simulink model "dfig(1)"  (R2022b)
settings: Solver=VariableStepAuto  StartTime=0.0  StopTime=10.0  RelTol=1e-3
values from neighbouring files (symbols this model uses):
  Cbus = 80e-3    (= 0.08)    [dfigcode.m]
  D = 1e-3    (= 0.001)    [dfigcode.m]
  f = 50    [dfigcode.m]
  Fs = Vs*sqrt(2/3)/(2*pi*f)    [dfigcode.m]
  fsw = 4e3    (= 4000)    [dfigcode.m]
  J = 127/2    (= 63.5)    [dfigcode.m]
  ki_id = (wni^2)*Lr*sigma    (= 491.599501999)    [dfigcode.m]
  Ki_idg = (wnig^2)*Lg    (= 56.8489213503)    [dfigcode.m]
  ki_iq = ki_id    (= 491.599501999)    [dfigcode.m]
  Ki_iqg = Ki_idg    (= 56.8489213503)    [dfigcode.m]
  ki_n = ((wnn^2)*J)/p    (= 12700)    [dfigcode.m]
  Ki_v = -300000    [dfigcode.m]
  Kopt = ((0.5*ro*pi*(Radio^5)*Cp_max)/(lambda_opt^3))    (= 296454.198186)    [dfigcode.m]
  kp_id = (2*wni*sigma*Lr)-Rr    (= 0.5771)    [dfigcode.m]
  Kp_idg = (2*wnig*Lg)-Rg    (= 0.301572894745)    [dfigcode.m]
  kp_iq = kp_id    (= 0.5771)    [dfigcode.m]
  Kp_iqg = Kp_idg    (= 0.301572894745)    [dfigcode.m]
  kp_n = (2*wnn*J)/p    (= 1270)    [dfigcode.m]
  Kp_v = -1000    [dfigcode.m]
  Kpg = 1/(1.5*Vs*sqrt(2/3))    [dfigcode.m]
  Kqg = -Kpg    [dfigcode.m]
  Lg = 400e-6    (= 0.0004)    [dfigcode.m]
  Lm = 2.5e-3    (= 0.0025)    [dfigcode.m]
  Ls = Lm + Lsi    (= 0.002587)    [dfigcode.m]
  Lsi = 0.087e-3    (= 8.7e-05)    [dfigcode.m]
  N = 100    [dfigcode.m]
  n = 1500    [dfigcode.m]
  p = 2    [dfigcode.m]
  Ps = 2e6    (= 2000000)    [dfigcode.m]
  Rg = 20e-6    (= 2e-05)    [dfigcode.m]
  Rr = 2.9e-3    (= 0.0029)    [dfigcode.m]
  Rs = 2.6e-3    (= 0.0026)    [dfigcode.m]
  smax = 1/3    (= 0.333333333333)    [dfigcode.m]
  tab_lambda = (0.1:0.01:11.8)    [dfigcode.m]
  Tem = 12732    [dfigcode.m]
  Ts = 1/fsw/50    (= 5e-06)    [dfigcode.m]
  Vbus = 1150    [dfigcode.m]
  Vs = 690    [dfigcode.m]
undefined symbols (not defined in the file or in its folder): Ct, DiscIntNeverNeededParam
libraries: spsSeriesRLCBranchLib x4, spsThreePhaseVIMeasurementLib x3, spsPWMGenerator2LevelLib x2, spsUniversalBridgeLib x2, spsAsynchronousMachineSIUnitsLib x1, spsGroundLib x1, spsMultimeterLib x1, spsThreePhaseProgrammableVoltageSourceLib x1, spsThreePhaseTransformerTwoWindingsLib x1, sps_lib x1
settings Model: Creator=prithika  LastModifiedBy=prithika

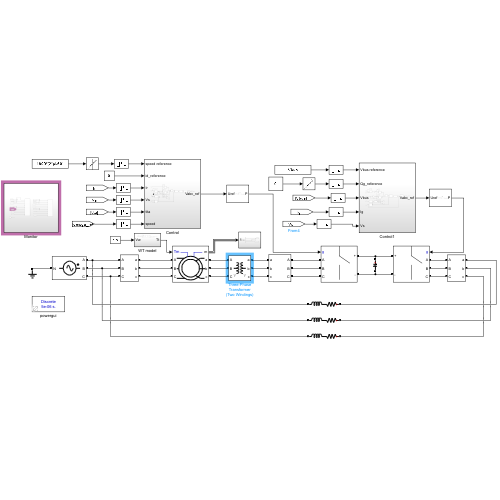
[thumbnail: Simulink's stored preview of the top-level diagram]
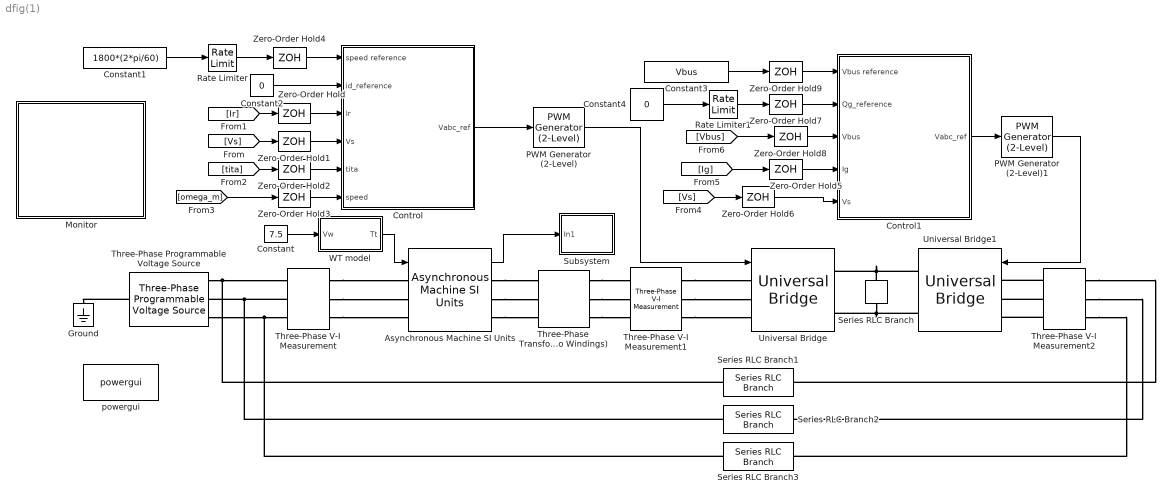
== system dfig(1) ==
  Asynchronous Machine SI Units : spsAsynchronousMachineSIUnitsLib/Asynchronous Machine SI Units  RotorType=Wound  PresetModel=No  MechanicalLoad=Torque Tm  ShowDetailedParameters=on  ReferenceFrame=Rotor  Units=SI  MeasurementBus=off  NominalParameters=[Ps Vs f]  VoltageRatio=1  Stator=[Rs , Lsi]  Rotor=[Rr , Lsi]  Cage1=[0.4155 0.002066]  Cage2=[0.4168 0.0003495]  Lm=Lm  Mechanical=[J D 2]  PolePairs=2  InitialConditions=[1 0 0 0 0 0 0 0]  SimulateSaturation=off  Saturation=[14.03593122, 27.81365428, 53.79336849, 72.68890987, 97.98006896, 148.6815601, 215.7428561, 302.9841135, 428.7778367 ; 230, 322, 414, 460, 506, 552, 598, 644, 690]  LoadFlowParameters=1492000  TsPowergui=0  TsBlock=-1  IterativeModel=Trapezoidal non iterative  IterativeDiscreteModel=Trapezoidal non iterative  Pmec=1.492e+006
  Constant : Constant  Value=7.5
  Constant1 : Constant  Value=1800*(2*pi/60)
  Constant2 : Constant  Value=0
  Constant3 : Constant  Value=Vbus
  Constant4 : Constant  Value=0
  Control : Subsystem
  Control1 : Subsystem
  Ground : spsGroundLib/Ground  LConnTagsString=a
  Monitor : Subsystem
  PWM Generator (2-Level) : spsPWMGenerator2LevelLib/PWM Generator (2-Level)  ModulatorType=Three-phase bridge (6 pulses)  ModulatorMode=Unsynchronized  Fc=fsw  Pc=0  nF=27  MinMax="[ -1  1 ]"  SamplingTechnique=Symmetrical regular (single edge)  ModulatingSignals=off  m=0.8  Freq=60  Phase=0  Ts=0  ShowCarrierOutport=off
  PWM Generator (2-Level)1 : spsPWMGenerator2LevelLib/PWM Generator (2-Level)  ModulatorType=Three-phase bridge (6 pulses)  ModulatorMode=Unsynchronized  Fc=fsw  Pc=0  nF=27  MinMax="[ -1  1 ]"  SamplingTechnique=Symmetrical regular (single edge)  ModulatingSignals=off  m=0.8  Freq=60  Phase=0  Ts=0  ShowCarrierOutport=off
  Rate Limiter : RateLimiter  RisingSlewLimit=100/1  FallingSlewLimit=-100/1  SampleTimeMode=inherited
  Rate Limiter1 : RateLimiter  RisingSlewLimit=1000e3/2  FallingSlewLimit=-1000e3/2  SampleTimeMode=inherited
  Series RLC Branch : spsSeriesRLCBranchLib/Series RLC Branch  LConnTagsString=__new0  RConnTagsString=__new0  BranchType=C  Resistance=1  Inductance=1e-3  SetiL0=off  InitialCurrent=0  Capacitance=Cbus  Setx0=on  InitialVoltage=0  Measurements=Branch voltage
  Series RLC Branch1 : spsSeriesRLCBranchLib/Series RLC Branch  LConnTagsString=__new0  RConnTagsString=__new0  BranchType=RL  Resistance=Rg  Inductance=Lg  SetiL0=off  InitialCurrent=0  Capacitance=Cbus  Setx0=on  InitialVoltage=0  Measurements=None
  Series RLC Branch2 : spsSeriesRLCBranchLib/Series RLC Branch  LConnTagsString=__new0  RConnTagsString=__new0  BranchType=RL  Resistance=Rg  Inductance=Lg  SetiL0=off  InitialCurrent=0  Capacitance=Cbus  Setx0=on  InitialVoltage=0  Measurements=None
  Series RLC Branch3 : spsSeriesRLCBranchLib/Series RLC Branch  LConnTagsString=__new0  RConnTagsString=__new0  BranchType=RL  Resistance=Rg  Inductance=Lg  SetiL0=off  InitialCurrent=0  Capacitance=Cbus  Setx0=on  InitialVoltage=0  Measurements=None
  Subsystem : Subsystem
  Three-Phase Programmable Voltage Source : spsThreePhaseProgrammableVoltageSourceLib/Three-Phase Programmable Voltage Source  PositiveSequence="[Vs  0 f]"  VariationEntity=None  VariationType=Table of time-amplitude pairs  VariationTypeAlt=Step  VariationStep=0.5  VariationRate=10  VariationMagnitude=0.3  VariationFrequency=2  VariationTiming=[1 2]  VariationPhaseA=off  Amplitudes=[1 0.8 1.2 1.0]  TimeValues=[0 0.1 0.15 0.2]  HarmonicGeneration=off  HarmonicA=[3 0.2 -25 0]  HarmonicB=[2 0.15 35 2]  Timing="[0.05  3]"  BusType=swing  Pref=0  Qref=0  Qmin=-inf  Qmax=inf
  Three-Phase Transformer (Two Windings) : spsThreePhaseTransformerTwoWindingsLib/Three-Phase Transformer (Two Windings)  Winding1Connection=Y  Winding2Connection=Y  CoreType=Three single-phase transformers  SetSaturation=off  Hysteresis=off  DataFile='hysteresis'  SetInitialFlux=off  Measurements=None  UNITS=SI  NominalPower=[ Ps , f ]  Winding1=[Vs 0 0]  Winding2=[Vs/u 0.0 0.0]  Rm=1.0804e+06  Lm=2866  L0=0.5  Saturation=[0 0;0.66653 1910.3;277.72 2419.7]  InitialFluxes=[ 0.8 , -0.8 , 0.7 ]  BreakLoop=off  DiscreteSolver=Trapezoidal iterative  DataType=on  TransfoNumber=1
  Three-Phase V-I Measurement : spsThreePhaseVIMeasurementLib/Three-Phase V-I Measurement  VoltageMeasurement=phase-to-ground  SetLabelV=on  LabelV=Vs  Vpu=off  VpuLL=off  CurrentMeasurement=yes  SetLabelI=on  LabelI=Is  Ipu=off  Pbase=100e6  Vbase=500e3  OutputType=Complex  PhasorSimulation=off  PSBequivalent=0
  Three-Phase V-I Measurement1 : spsThreePhaseVIMeasurementLib/Three-Phase V-I Measurement  VoltageMeasurement=no  SetLabelV=off  LabelV=Vs  Vpu=off  VpuLL=off  CurrentMeasurement=yes  SetLabelI=on  LabelI=Ir  Ipu=off  Pbase=100e6  Vbase=500e3  OutputType=Complex  PhasorSimulation=off  PSBequivalent=0
  Three-Phase V-I Measurement2 : spsThreePhaseVIMeasurementLib/Three-Phase V-I Measurement  VoltageMeasurement=no  SetLabelV=on  LabelV=Vs  Vpu=on  VpuLL=off  CurrentMeasurement=yes  SetLabelI=on  LabelI=Ig  Ipu=off  Pbase=100e6  Vbase=500e3  OutputType=Complex  PhasorSimulation=off  PSBequivalent=0
  Universal Bridge : spsUniversalBridgeLib/Universal Bridge  Arms=3  SnubberResistance=1e5  SnubberCapacitance=inf  Device=Ideal Switches  Ron=1e-3  Lon=0  ForwardVoltages="[  0  0  ]"  ForwardVoltage=0  GTOparameters=[ 10e-6 , 20e-6 ]  IGBTparameters=[ 1e-6 , 2e-6 ]  Measurements=None  Measurements_2=None  converterType=Rectifier
  Universal Bridge1 : spsUniversalBridgeLib/Universal Bridge  Arms=3  SnubberResistance=1e5  SnubberCapacitance=inf  Device=Ideal Switches  Ron=1e-3  Lon=0  ForwardVoltages="[  0  0  ]"  ForwardVoltage=0  GTOparameters=[ 10e-6 , 20e-6 ]  IGBTparameters=[ 1e-6 , 2e-6 ]  Measurements=None  Measurements_2=None  converterType=Rectifier
  WT model : Subsystem
  Zero-Order Hold{,1..9} (10 alike) : ZeroOrderHold  SampleTime=1/fsw
  powergui : sps_lib/powergui  Priority=1  SimulationMode=Discrete  SampleTime=Ts  frequency=60  Iterations=50  frequencyindice=50  Pbase=100e6  ErrMax=1e-4  UnitsV=kV  UnitsW=MW  buscounter=0  FunctionMessages=off  echomessages=off  EnableUseOfTLC=off  CurrentSourceSwitches=off  DisableSnubberDevices=off  DisableRonSwitches=off  DisableVfSwitches=off  DisplayEquations=off  AutomaticDiscreteSolvers=off  SolverType=Tustin/Backward Euler (TBE)  Interpol=off  ExternalGateDelay=off  methode=off  Ts=100  x0status=blocks  SPID=on  SwTol=0  HookPort=off  NonlinearTolerance=1e-4  nMaxIteration=100  ContinueOnMaxIteration=off  RestoreLinks=warning  ResistiveCurrentMeasurement=off  Frange=[0:2:500]  Ylog=off  Xlog=on  ShowGrid=off  save=off  variable=ZData  structure=0  ZoomFFT=off  StartTime=0.0  cycles=1  DisplayStyle=1  fundamental=60  FreqAxis=off  MaxFrequency=1000  frequencyindicesteady=1  RmsSteady=1  display=off
  wires:
  PWM Generator (2-Level)/1 -> Universal Bridge/1
  Control/1(Vabc_ref) -> PWM Generator (2-Level)/1
  Constant2/1 -> Control/2(id_reference)
  Constant1/1 -> Rate Limiter/1
  [Vs] -> Zero-Order Hold1/1
  [Ir] -> Zero-Order Hold/1
  Asynchronous Machine SI Units/1 -> Subsystem/1(In1)
  [tita] -> Zero-Order Hold2/1
  [omega_m] -> Zero-Order Hold3/1
  Zero-Order Hold/1 -> Control/3(Ir)
  Zero-Order Hold1/1 -> Control/4(Vs)
  Zero-Order Hold2/1 -> Control/5(tita)
  Zero-Order Hold3/1 -> Control/6(speed)
  Zero-Order Hold4/1 -> Control/1(speed reference)
  Rate Limiter/1 -> Zero-Order Hold4/1
  Constant/1 -> WT model/1(Vw)
  WT model/1(Tt) -> Asynchronous Machine SI Units/1
  PWM Generator (2-Level)1/1 -> Universal Bridge1/1
  Constant4/1 -> Rate Limiter1/1
  Zero-Order Hold9/1 -> Control1/1(Vbus reference)
  Constant3/1 -> Zero-Order Hold9/1
  [Vs] -> Zero-Order Hold6/1
  [Ig] -> Zero-Order Hold5/1
  Zero-Order Hold5/1 -> Control1/4(Ig)
  Zero-Order Hold6/1 -> Control1/5(Vs)
  Control1/1(Vabc_ref) -> PWM Generator (2-Level)1/1
  Zero-Order Hold7/1 -> Control1/2(Qg_reference)
  Rate Limiter1/1 -> Zero-Order Hold7/1
  [Vbus] -> Zero-Order Hold8/1
  Zero-Order Hold8/1 -> Control1/3(Vbus)
  connections:
  Three-Phase Programmable Voltage Source/LConn1 -- Ground/LConn1
  Three-Phase V-I Measurement1/LConn2 -- Universal Bridge/LConn2
  Three-Phase V-I Measurement1/LConn1 -- Universal Bridge/LConn1
  Three-Phase V-I Measurement1/LConn3 -- Universal Bridge/LConn3
  Three-Phase Programmable Voltage Source/RConn1 -- Series RLC Branch1/RConn1 -- Three-Phase V-I Measurement/LConn1
  Three-Phase V-I Measurement/LConn2 -- Series RLC Branch2/RConn1 -- Three-Phase Programmable Voltage Source/RConn2
  Three-Phase Programmable Voltage Source/RConn3 -- Series RLC Branch3/RConn1 -- Three-Phase V-I Measurement/LConn3
  Three-Phase V-I Measurement/RConn1 -- Asynchronous Machine SI Units/LConn1
  Three-Phase V-I Measurement/RConn2 -- Asynchronous Machine SI Units/LConn2
  Three-Phase V-I Measurement/RConn3 -- Asynchronous Machine SI Units/LConn3
  Universal Bridge1/RConn1 -- Series RLC Branch/LConn1 -- Universal Bridge/RConn1
  Universal Bridge1/RConn2 -- Series RLC Branch/RConn1 -- Universal Bridge/RConn2
  Three-Phase V-I Measurement2/LConn2 -- Universal Bridge1/LConn2
  Three-Phase V-I Measurement2/LConn1 -- Universal Bridge1/LConn1
  Three-Phase V-I Measurement2/LConn3 -- Universal Bridge1/LConn3
  Three-Phase V-I Measurement2/RConn1 -- Series RLC Branch1/LConn1
  Three-Phase V-I Measurement2/RConn2 -- Series RLC Branch2/LConn1
  Three-Phase V-I Measurement2/RConn3 -- Series RLC Branch3/LConn1
  Asynchronous Machine SI Units/RConn1 -- Three-Phase Transformer (Two Windings)/LConn1
  Three-Phase Transformer (Two Windings)/RConn1 -- Three-Phase V-I Measurement1/RConn1
  Asynchronous Machine SI Units/RConn2 -- Three-Phase Transformer (Two Windings)/LConn2
  Asynchronous Machine SI Units/RConn3 -- Three-Phase Transformer (Two Windings)/LConn3
  Three-Phase Transformer (Two Windings)/RConn2 -- Three-Phase V-I Measurement1/RConn2
  Three-Phase Transformer (Two Windings)/RConn3 -- Three-Phase V-I Measurement1/RConn3

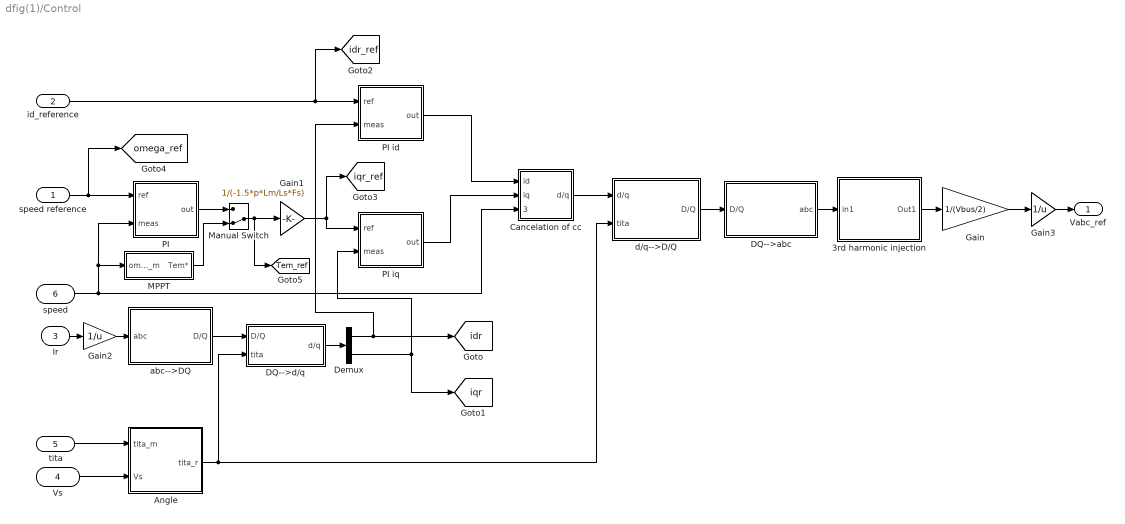
== system dfig(1)/Control ==
  speed reference : Inport
  id_reference : Inport  Port=2
  Ir : Inport  Port=3
  Vs : Inport  Port=4
  tita : Inport  Port=5
  speed : Inport  Port=6
  3rd harmonic injection : Subsystem
  Angle : Subsystem
  Cancelation of cc : Subsystem
  DQ-->abc : Subsystem
  DQ-->d/q : Subsystem
  Demux : Demux  Outputs=2
  Gain : Gain  Gain=1/(Vbus/2)
  Gain1 : Gain  Gain=1/(-1.5*p*Lm/Ls*Fs)
  Gain2 : Gain  Gain=1/u
  Gain3 : Gain  Gain=1/u
  MPPT : Subsystem
  Manual Switch : ManualSwitch  CurrentSetting=0
  "PI " : Subsystem
  PI id : Subsystem
  PI iq : Subsystem
  abc-->DQ : Subsystem
  d/q-->D/Q : Subsystem
  Vabc_ref : Outport
  tag scope: Tem_ref=global, idr=global, idr_ref=global, iqr=global, iqr_ref=global, omega_ref=global
  wires:
  DQ-->abc/1(abc) -> 3rd harmonic injection/1(in1)
  d/q-->D/Q/1(D/Q) -> DQ-->abc/1(D/Q)
  abc-->DQ/1(D/Q) -> DQ-->d/q/1(D/Q)
  3rd harmonic injection/1(Out1) -> Gain/1
  tita/1 -> Angle/1(tita_m)
  Vs/1 -> Angle/2(Vs)
  Angle/1(tita_r) -> d/q-->D/Q/2(tita), DQ-->d/q/2(tita)
  Cancelation of cc/1(d/q) -> d/q-->D/Q/1(d/q)
  PI id/1(out) -> Cancelation of cc/1(id)
  PI iq/1(out) -> Cancelation of cc/2(iq)
  speed/1 -> MPPT/1(omega_m), "PI "/2(meas), Cancelation of cc/3(omega)
  DQ-->d/q/1(d/q) -> Demux/1
  Demux/2 -> [iqr], PI iq/2(meas)
  Demux/1 -> [idr], PI id/2(meas)
  speed reference/1 -> [omega_ref], "PI "/1(ref)
  Gain1/1 -> [iqr_ref], PI iq/1(ref)
  id_reference/1 -> PI id/1(ref), [idr_ref]
  MPPT/1(Tem*) -> Manual Switch/2
  "PI "/1(out) -> Manual Switch/1
  Manual Switch/1 -> Gain1/1, [Tem_ref]
  Ir/1 -> Gain2/1
  Gain2/1 -> abc-->DQ/1(abc)
  Gain/1 -> Gain3/1
  Gain3/1 -> Vabc_ref/1

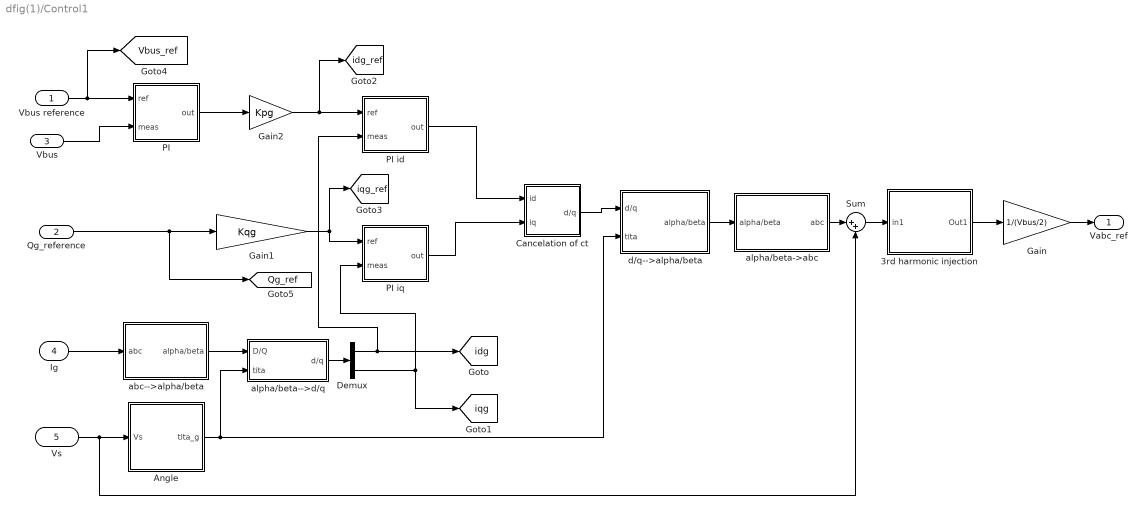
== system dfig(1)/Control1 ==
  Vbus reference : Inport
  Qg_reference : Inport  Port=2
  Vbus : Inport  Port=3
  Ig : Inport  Port=4
  Vs : Inport  Port=5
  3rd harmonic injection : Subsystem
  Angle : Subsystem
  Cancelation of ct : Subsystem
  Demux : Demux  Outputs=2
  Gain : Gain  Gain=1/(Vbus/2)
  Gain1 : Gain  Gain=Kqg
  Gain2 : Gain  Gain=Kpg
  "PI " : Subsystem
  PI id : Subsystem
  PI iq : Subsystem
  Sum : Sum  Inputs=|++
  abc-->alpha/beta : Subsystem
  alpha/beta-->d/q : Subsystem
  alpha/beta->abc : Subsystem
  d/q-->alpha/beta : Subsystem
  Vabc_ref : Outport
  tag scope: Qg_ref=global, Vbus_ref=global, idg=global, idg_ref=global, iqg=global, iqg_ref=global
  wires:
  Gain/1 -> Vabc_ref/1
  d/q-->alpha/beta/1(alpha/beta) -> alpha/beta->abc/1(alpha/beta)
  Ig/1 -> abc-->alpha/beta/1(abc)
  abc-->alpha/beta/1(alpha/beta) -> alpha/beta-->d/q/1(D/Q)
  3rd harmonic injection/1(Out1) -> Gain/1
  Vs/1 -> Sum/2, Angle/1(Vs)
  Angle/1(tita_g) -> d/q-->alpha/beta/2(tita), alpha/beta-->d/q/2(tita)
  Cancelation of ct/1(d/q) -> d/q-->alpha/beta/1(d/q)
  PI id/1(out) -> Cancelation of ct/1(id)
  PI iq/1(out) -> Cancelation of ct/2(iq)
  alpha/beta-->d/q/1(d/q) -> Demux/1
  Demux/2 -> [iqg], PI iq/2(meas)
  Demux/1 -> [idg], PI id/2(meas)
  Vbus reference/1 -> "PI "/1(ref), [Vbus_ref]
  Gain1/1 -> [iqg_ref], PI iq/1(ref)
  Qg_reference/1 -> Gain1/1, [Qg_ref]
  "PI "/1(out) -> Gain2/1
  Gain2/1 -> [idg_ref], PI id/1(ref)
  Vbus/1 -> "PI "/2(meas)
  alpha/beta->abc/1(abc) -> Sum/1
  Sum/1 -> 3rd harmonic injection/1(in1)

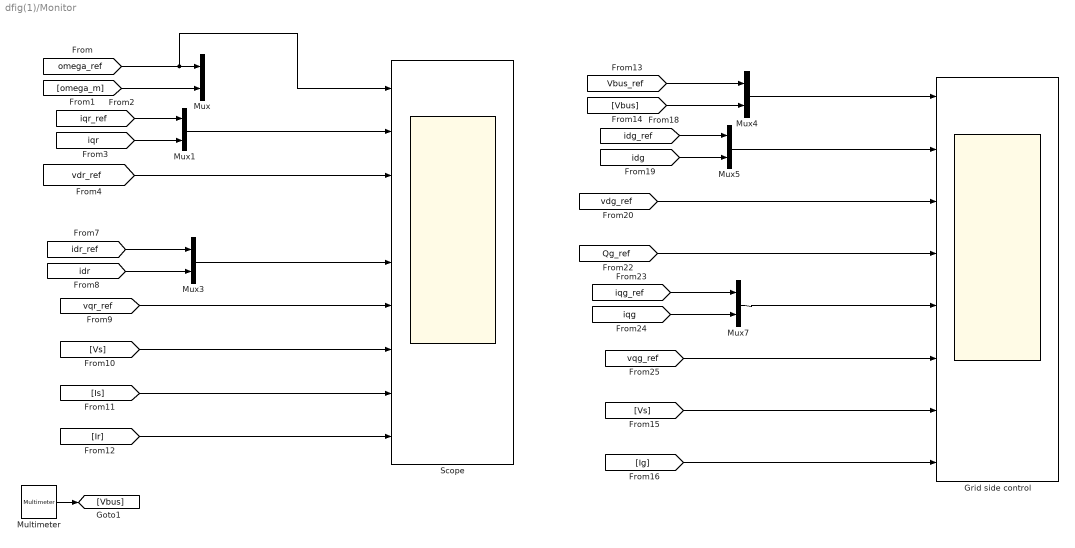
== system dfig(1)/Monitor ==
  Grid side control : Scope  NumInputPorts=8
  Multimeter : spsMultimeterLib/Multimeter  L=1  sel=1  yselected={}  Gain=0  OutputType=Complex  PlotAtSimulationStop=off  PhasorSimulation=off
  Mux{,1,3..5,7} (6 alike) : Mux  Inputs=2
  Scope : Scope  NumInputPorts=9
  wires:
  [omega_ref] -> Scope/1, Mux/1
  [omega_m] -> Mux/2
  [iqr_ref] -> Mux1/1
  [iqr] -> Mux1/2
  Mux1/1 -> Scope/2
  [vdr_ref] -> Scope/3
  [idr_ref] -> Mux3/1
  [idr] -> Mux3/2
  Mux3/1 -> Scope/5
  [Vs] -> Scope/7
  [Is] -> Scope/8
  [Ir] -> Scope/9
  [vqr_ref] -> Scope/6
  Multimeter/1 -> [Vbus]
  [Qg_ref] -> Grid side control/4
  [vqg_ref] -> Grid side control/6
  [vdg_ref] -> Grid side control/3
  [iqg] -> Mux7/2
  [iqg_ref] -> Mux7/1
  [Vbus_ref] -> Mux4/1
  [Vbus] -> Mux4/2
  [Ig] -> Grid side control/8
  [Vs] -> Grid side control/7
  Mux5/1 -> Grid side control/2
  [idg_ref] -> Mux5/1
  [idg] -> Mux5/2
  Mux7/1 -> Grid side control/5
  Mux4/1 -> Grid side control/1

== system dfig(1)/Subsystem ==
  In1 : Inport
  Bus Selector : BusSelector  OutputSignals=Mechanical.Rotor angle thetam (rad),Mechanical.Rotor speed (wm),Mechanical.Electromagnetic torque Te (N*m)
  wires:
  In1/1 -> Bus Selector/1
  Bus Selector/2 -> [omega_m]  "<Rotor speed (wm)>"
  Bus Selector/1 -> [tita]  "<Rotor angle thetam (rad)>"
  Bus Selector/3 -> [Tem]  "<Electromagnetic torque Te (N*m)>"

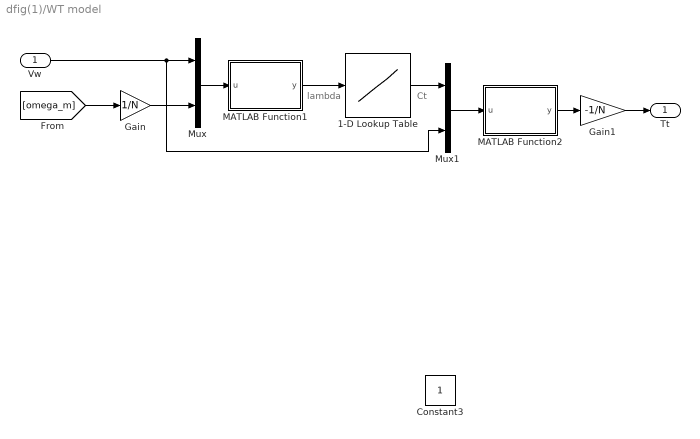
== system dfig(1)/WT model ==
  note: Ct
  note: lambda
  Vw : Inport
  1-D Lookup Table : Lookup_n-D  NumberOfTableDimensions=1  BreakpointsForDimension1=tab_lambda  BreakpointsForDimension1DataTypeStr=Inherit: Inherit from 'Breakpoint data'  Table=Ct  TableDataTypeStr=Inherit: Inherit from 'Table data'  InternalRulePriority=Speed  RndMeth=Simplest
  Constant3 : Constant
  Gain : Gain  Gain=1/N
  Gain1 : Gain  Gain=-1/N
  MATLAB Function1 : MATLAB Function  TreatAsAtomicUnit=on
  MATLAB Function2 : MATLAB Function  TreatAsAtomicUnit=on
  Mux : Mux  Inputs=2
  Mux1 : Mux  Inputs=2
  Tt : Outport
  wires:
  Vw/1 -> Mux1/2, Mux/1
  [omega_m] -> Gain/1
  Gain/1 -> Mux/2
  Mux/1 -> MATLAB Function1/1(u)
  MATLAB Function1/1(y) -> 1-D Lookup Table/1
  MATLAB Function2/1(y) -> Gain1/1
  Gain1/1 -> Tt/1
  1-D Lookup Table/1 -> Mux1/1
  Mux1/1 -> MATLAB Function2/1(u)

== system dfig(1)/Control/3rd harmonic injection ==
  in1 : Inport
  Gain : Gain  Gain=-0.5
  Max1 : MinMax  Function=max
  Min1 : MinMax
  Sum : Sum  Inputs=|++
  Sum1 : Sum  Inputs=|++
  Out1 : Outport
  wires:
  in1/1 -> Max1/1, Min1/1, Sum/1
  Sum/1 -> Out1/1
  Min1/1 -> Sum1/1
  Sum1/1 -> Gain/1
  Gain/1 -> Sum/2
  Max1/1 -> Sum1/2

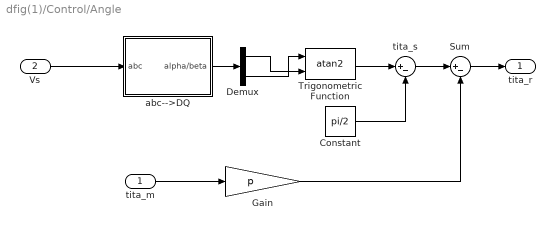
== system dfig(1)/Control/Angle ==
  tita_m : Inport
  Vs : Inport  Port=2
  Constant : Constant  Value=pi/2
  Demux : Demux  Outputs=2
  Gain : Gain  Gain=p
  Sum : Sum  Inputs=|+-
  Trigonometric Function : Trigonometry  Operator=atan2
  abc-->DQ : Subsystem
  tita_s : Sum  Inputs=|+-
  tita_r : Outport
  wires:
  Vs/1 -> abc-->DQ/1(abc)
  abc-->DQ/1(alpha/beta) -> Demux/1
  Demux/1 -> Trigonometric Function/2
  Demux/2 -> Trigonometric Function/1
  Trigonometric Function/1 -> tita_s/1
  Constant/1 -> tita_s/2
  tita_m/1 -> Gain/1
  tita_s/1 -> Sum/1
  Sum/1 -> tita_r/1
  Gain/1 -> Sum/2

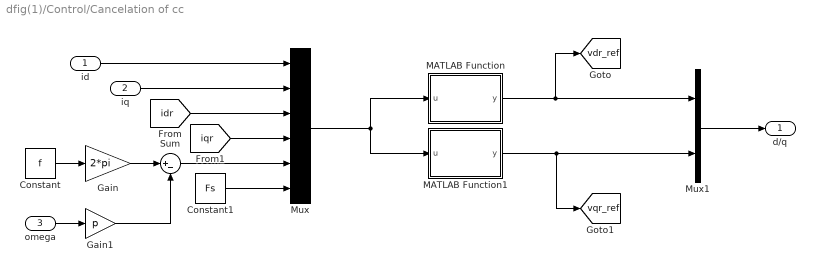
== system dfig(1)/Control/Cancelation of cc ==
  id : Inport
  iq : Inport  Port=2
  omega : Inport  Port=3
  Constant : Constant  Value=f
  Constant1 : Constant  Value=Fs
  Gain : Gain  Gain=2*pi
  Gain1 : Gain  Gain=p
  MATLAB Function : MATLAB Function  TreatAsAtomicUnit=on
  MATLAB Function1 : MATLAB Function  TreatAsAtomicUnit=on
  Mux : Mux  Inputs=6
  Mux1 : Mux  Inputs=2
  Sum : Sum  Inputs=|+-
  d/q : Outport
  tag scope: vdr_ref=global, vqr_ref=global
  wires:
  id/1 -> Mux/1
  iq/1 -> Mux/2
  [idr] -> Mux/3
  [iqr] -> Mux/4
  Constant/1 -> Gain/1
  Gain/1 -> Sum/1
  Sum/1 -> Mux/5
  Constant1/1 -> Mux/6
  omega/1 -> Gain1/1
  Gain1/1 -> Sum/2
  Mux/1 -> MATLAB Function/1(u), MATLAB Function1/1(u)
  MATLAB Function/1(y) -> [vdr_ref], Mux1/1
  MATLAB Function1/1(y) -> [vqr_ref], Mux1/2
  Mux1/1 -> d/q/1

== system dfig(1)/Control/DQ-->abc ==
  D/Q : Inport
  MATLAB Function : MATLAB Function  TreatAsAtomicUnit=on
  MATLAB Function1 : MATLAB Function  TreatAsAtomicUnit=on
  MATLAB Function2 : MATLAB Function  TreatAsAtomicUnit=on
  Mux : Mux  Inputs=3
  abc : Outport
  wires:
  MATLAB Function/1(y) -> Mux/1
  MATLAB Function1/1(y) -> Mux/2
  MATLAB Function2/1(y) -> Mux/3
  D/Q/1 -> MATLAB Function2/1(u), MATLAB Function1/1(u), MATLAB Function/1(u)
  Mux/1 -> abc/1

== system dfig(1)/Control/DQ-->d//q ==
  D/Q : Inport
  tita : Inport  Port=2
  MATLAB Function : MATLAB Function  TreatAsAtomicUnit=on
  MATLAB Function1 : MATLAB Function  TreatAsAtomicUnit=on
  Mux : Mux  Inputs=2
  Mux1 : Mux  Inputs=2
  d/q : Outport
  wires:
  D/Q/1 -> Mux/1
  tita/1 -> Mux/2
  Mux/1 -> MATLAB Function1/1(u), MATLAB Function/1(u)
  MATLAB Function/1(y) -> Mux1/1
  MATLAB Function1/1(y) -> Mux1/2
  Mux1/1 -> d/q/1

== system dfig(1)/Control/MPPT ==
  omega_m : Inport
  Gain : Gain  Gain=1/N
  Gain1 : Gain  Gain=-Kopt
  Gain2 : Gain  Gain=1/n
  MATLAB Function : MATLAB Function  TreatAsAtomicUnit=on
  Tem* : Outport
  wires:
  MATLAB Function/1(y) -> Gain1/1
  omega_m/1 -> Gain/1
  Gain/1 -> MATLAB Function/1(u)
  Gain1/1 -> Gain2/1
  Gain2/1 -> Tem*/1

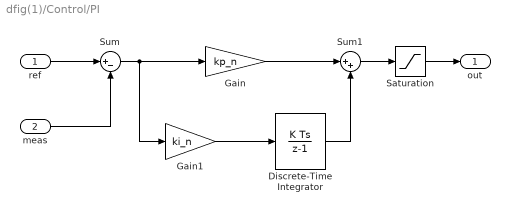
== system dfig(1)/Control/PI  ==
  ref : Inport
  meas : Inport  Port=2
  Discrete-Time Integrator : DiscreteIntegrator  SampleTime=1/fsw  LimitOutput=on  UpperSaturationLimit=Tem  LowerSaturationLimit=-Tem  ICPrevOutput=DiscIntNeverNeededParam  ICPrevScaledInput=DiscIntNeverNeededParam
  Gain : Gain  Gain=kp_n
  Gain1 : Gain  Gain=ki_n
  Saturation : Saturate  UpperLimit=Tem  LowerLimit=-Tem
  Sum : Sum  Inputs=|+-
  Sum1 : Sum  Inputs=|++
  out : Outport
  wires:
  Gain1/1 -> Discrete-Time Integrator/1
  Sum1/1 -> Saturation/1
  ref/1 -> Sum/1
  meas/1 -> Sum/2
  Sum/1 -> Gain1/1, Gain/1
  Gain/1 -> Sum1/1
  Discrete-Time Integrator/1 -> Sum1/2
  Saturation/1 -> out/1

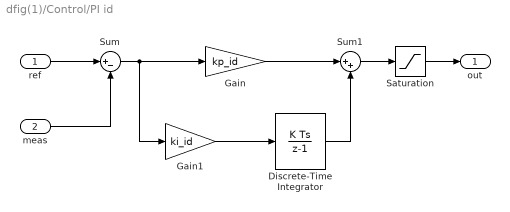
== system dfig(1)/Control/PI id ==
  ref : Inport
  meas : Inport  Port=2
  Discrete-Time Integrator : DiscreteIntegrator  SampleTime=1/fsw  LimitOutput=on  UpperSaturationLimit=Vbus/sqrt(3)  LowerSaturationLimit=-Vbus/sqrt(3)  ICPrevOutput=DiscIntNeverNeededParam  ICPrevScaledInput=DiscIntNeverNeededParam
  Gain : Gain  Gain=kp_id
  Gain1 : Gain  Gain=ki_id
  Saturation : Saturate  UpperLimit=Vbus/sqrt(3)  LowerLimit=-Vbus/sqrt(3)
  Sum : Sum  Inputs=|+-
  Sum1 : Sum  Inputs=|++
  out : Outport
  wires:
  Gain1/1 -> Discrete-Time Integrator/1
  Sum1/1 -> Saturation/1
  ref/1 -> Sum/1
  meas/1 -> Sum/2
  Sum/1 -> Gain1/1, Gain/1
  Gain/1 -> Sum1/1
  Discrete-Time Integrator/1 -> Sum1/2
  Saturation/1 -> out/1

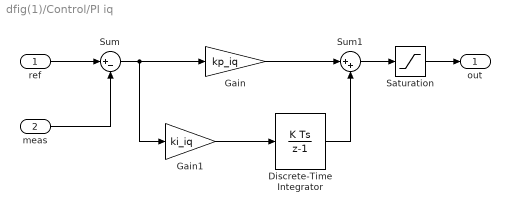
== system dfig(1)/Control/PI iq ==
  ref : Inport
  meas : Inport  Port=2
  Discrete-Time Integrator : DiscreteIntegrator  SampleTime=1/fsw  LimitOutput=on  UpperSaturationLimit=Vbus/sqrt(3)  LowerSaturationLimit=-Vbus/sqrt(3)  ICPrevOutput=DiscIntNeverNeededParam  ICPrevScaledInput=DiscIntNeverNeededParam
  Gain : Gain  Gain=kp_iq
  Gain1 : Gain  Gain=ki_iq
  Saturation : Saturate  UpperLimit=Vbus/sqrt(3)  LowerLimit=-Vbus/sqrt(3)
  Sum : Sum  Inputs=|+-
  Sum1 : Sum  Inputs=|++
  out : Outport
  wires:
  Gain1/1 -> Discrete-Time Integrator/1
  Sum1/1 -> Saturation/1
  ref/1 -> Sum/1
  meas/1 -> Sum/2
  Sum/1 -> Gain1/1, Gain/1
  Gain/1 -> Sum1/1
  Discrete-Time Integrator/1 -> Sum1/2
  Saturation/1 -> out/1

== system dfig(1)/Control/abc-->DQ ==
  abc : Inport
  MATLAB Function : MATLAB Function  TreatAsAtomicUnit=on
  MATLAB Function1 : MATLAB Function  TreatAsAtomicUnit=on
  Mux : Mux  Inputs=2
  D/Q : Outport
  wires:
  abc/1 -> MATLAB Function1/1(u), MATLAB Function/1(u)
  MATLAB Function/1(y) -> Mux/1
  MATLAB Function1/1(y) -> Mux/2
  Mux/1 -> D/Q/1

== system dfig(1)/Control/d//q-->D//Q ==
  d/q : Inport
  tita : Inport  Port=2
  MATLAB Function : MATLAB Function  TreatAsAtomicUnit=on
  MATLAB Function1 : MATLAB Function  TreatAsAtomicUnit=on
  Mux : Mux  Inputs=2
  Mux1 : Mux  Inputs=2
  D/Q : Outport
  wires:
  d/q/1 -> Mux/1
  tita/1 -> Mux/2
  Mux/1 -> MATLAB Function1/1(u), MATLAB Function/1(u)
  MATLAB Function/1(y) -> Mux1/1
  MATLAB Function1/1(y) -> Mux1/2
  Mux1/1 -> D/Q/1

== system dfig(1)/Control1/3rd harmonic injection ==
  in1 : Inport
  Gain : Gain  Gain=-0.5
  Max1 : MinMax  Function=max
  Min1 : MinMax
  Sum : Sum  Inputs=|++
  Sum1 : Sum  Inputs=|++
  Out1 : Outport
  wires:
  in1/1 -> Max1/1, Min1/1, Sum/1
  Sum/1 -> Out1/1
  Min1/1 -> Sum1/1
  Sum1/1 -> Gain/1
  Gain/1 -> Sum/2
  Max1/1 -> Sum1/2

== system dfig(1)/Control1/Angle ==
  note: tita_g
  Vs : Inport
  Demux : Demux  Outputs=2
  Trigonometric Function : Trigonometry  Operator=atan2
  abc-->alpha/beta : Subsystem
  tita_g : Outport
  wires:
  Vs/1 -> abc-->alpha/beta/1(abc)
  abc-->alpha/beta/1(alpha/beta) -> Demux/1
  Demux/1 -> Trigonometric Function/2
  Demux/2 -> Trigonometric Function/1
  Trigonometric Function/1 -> tita_g/1

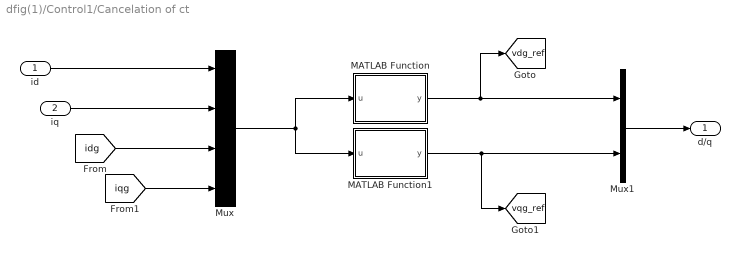
== system dfig(1)/Control1/Cancelation of ct ==
  id : Inport
  iq : Inport  Port=2
  MATLAB Function : MATLAB Function  TreatAsAtomicUnit=on
  MATLAB Function1 : MATLAB Function  TreatAsAtomicUnit=on
  Mux : Mux
  Mux1 : Mux  Inputs=2
  d/q : Outport
  tag scope: vdg_ref=global, vqg_ref=global
  wires:
  id/1 -> Mux/1
  iq/1 -> Mux/2
  [idg] -> Mux/3
  [iqg] -> Mux/4
  Mux/1 -> MATLAB Function/1(u), MATLAB Function1/1(u)
  MATLAB Function/1(y) -> [vdg_ref], Mux1/1
  MATLAB Function1/1(y) -> [vqg_ref], Mux1/2
  Mux1/1 -> d/q/1

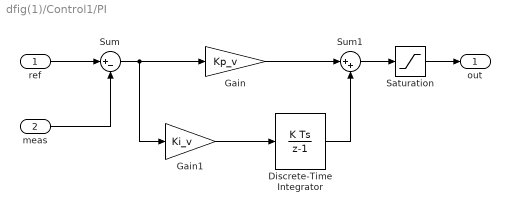
== system dfig(1)/Control1/PI  ==
  ref : Inport
  meas : Inport  Port=2
  Discrete-Time Integrator : DiscreteIntegrator  SampleTime=1/fsw  LimitOutput=on  UpperSaturationLimit=Ps*smax  LowerSaturationLimit=-Ps*smax  ICPrevOutput=DiscIntNeverNeededParam  ICPrevScaledInput=DiscIntNeverNeededParam
  Gain : Gain  Gain=Kp_v
  Gain1 : Gain  Gain=Ki_v
  Saturation : Saturate  UpperLimit=Ps*smax  LowerLimit=-Ps*smax
  Sum : Sum  Inputs=|+-
  Sum1 : Sum  Inputs=|++
  out : Outport
  wires:
  Gain1/1 -> Discrete-Time Integrator/1
  Sum1/1 -> Saturation/1
  ref/1 -> Sum/1
  meas/1 -> Sum/2
  Sum/1 -> Gain1/1, Gain/1
  Gain/1 -> Sum1/1
  Discrete-Time Integrator/1 -> Sum1/2
  Saturation/1 -> out/1

== system dfig(1)/Control1/PI id ==
  ref : Inport
  meas : Inport  Port=2
  Discrete-Time Integrator : DiscreteIntegrator  SampleTime=1/fsw  LimitOutput=on  UpperSaturationLimit=Vbus/sqrt(3)  LowerSaturationLimit=-Vbus/sqrt(3)  ICPrevOutput=DiscIntNeverNeededParam  ICPrevScaledInput=DiscIntNeverNeededParam
  Gain : Gain  Gain=Kp_idg
  Gain1 : Gain  Gain=Ki_idg
  Saturation : Saturate  UpperLimit=Vbus/sqrt(3)  LowerLimit=-Vbus/sqrt(3)
  Sum : Sum  Inputs=|+-
  Sum1 : Sum  Inputs=|++
  out : Outport
  wires:
  Gain1/1 -> Discrete-Time Integrator/1
  Sum1/1 -> Saturation/1
  ref/1 -> Sum/1
  meas/1 -> Sum/2
  Sum/1 -> Gain1/1, Gain/1
  Gain/1 -> Sum1/1
  Discrete-Time Integrator/1 -> Sum1/2
  Saturation/1 -> out/1

== system dfig(1)/Control1/PI iq ==
  ref : Inport
  meas : Inport  Port=2
  Discrete-Time Integrator : DiscreteIntegrator  SampleTime=1/fsw  LimitOutput=on  UpperSaturationLimit=Vbus/sqrt(3)  LowerSaturationLimit=-Vbus/sqrt(3)  ICPrevOutput=DiscIntNeverNeededParam  ICPrevScaledInput=DiscIntNeverNeededParam
  Gain : Gain  Gain=Kp_iqg
  Gain1 : Gain  Gain=Ki_iqg
  Saturation : Saturate  UpperLimit=Vbus/sqrt(3)  LowerLimit=-Vbus/sqrt(3)
  Sum : Sum  Inputs=|+-
  Sum1 : Sum  Inputs=|++
  out : Outport
  wires:
  Gain1/1 -> Discrete-Time Integrator/1
  Sum1/1 -> Saturation/1
  ref/1 -> Sum/1
  meas/1 -> Sum/2
  Sum/1 -> Gain1/1, Gain/1
  Gain/1 -> Sum1/1
  Discrete-Time Integrator/1 -> Sum1/2
  Saturation/1 -> out/1

== system dfig(1)/Control1/abc-->alpha//beta ==
  abc : Inport
  MATLAB Function : MATLAB Function  TreatAsAtomicUnit=on
  MATLAB Function1 : MATLAB Function  TreatAsAtomicUnit=on
  Mux : Mux  Inputs=2
  alpha/beta : Outport
  wires:
  abc/1 -> MATLAB Function1/1(u), MATLAB Function/1(u)
  MATLAB Function/1(y) -> Mux/1
  MATLAB Function1/1(y) -> Mux/2
  Mux/1 -> alpha/beta/1

== system dfig(1)/Control1/alpha//beta-->d//q ==
  D/Q : Inport
  tita : Inport  Port=2
  MATLAB Function : MATLAB Function  TreatAsAtomicUnit=on
  MATLAB Function1 : MATLAB Function  TreatAsAtomicUnit=on
  Mux : Mux  Inputs=2
  Mux1 : Mux  Inputs=2
  d/q : Outport
  wires:
  D/Q/1 -> Mux/1
  tita/1 -> Mux/2
  Mux/1 -> MATLAB Function1/1(u), MATLAB Function/1(u)
  MATLAB Function/1(y) -> Mux1/1
  MATLAB Function1/1(y) -> Mux1/2
  Mux1/1 -> d/q/1

== system dfig(1)/Control1/alpha//beta->abc ==
  alpha/beta : Inport
  MATLAB Function : MATLAB Function  TreatAsAtomicUnit=on
  MATLAB Function1 : MATLAB Function  TreatAsAtomicUnit=on
  MATLAB Function2 : MATLAB Function  TreatAsAtomicUnit=on
  Mux : Mux  Inputs=3
  abc : Outport
  wires:
  MATLAB Function/1(y) -> Mux/1
  MATLAB Function1/1(y) -> Mux/2
  MATLAB Function2/1(y) -> Mux/3
  alpha/beta/1 -> MATLAB Function2/1(u), MATLAB Function1/1(u), MATLAB Function/1(u)
  Mux/1 -> abc/1

== system dfig(1)/Control1/d//q-->alpha//beta ==
  d/q : Inport
  tita : Inport  Port=2
  MATLAB Function : MATLAB Function  TreatAsAtomicUnit=on
  MATLAB Function1 : MATLAB Function  TreatAsAtomicUnit=on
  Mux : Mux  Inputs=2
  Mux1 : Mux  Inputs=2
  alpha/beta : Outport
  wires:
  d/q/1 -> Mux/1
  tita/1 -> Mux/2
  Mux/1 -> MATLAB Function1/1(u), MATLAB Function/1(u)
  MATLAB Function/1(y) -> Mux1/1
  MATLAB Function1/1(y) -> Mux1/2
  Mux1/1 -> alpha/beta/1

== system dfig(1)/Control/Angle/abc-->DQ ==
  abc : Inport
  MATLAB Function : MATLAB Function  TreatAsAtomicUnit=on
  MATLAB Function1 : MATLAB Function  TreatAsAtomicUnit=on
  Mux : Mux  Inputs=2
  alpha/beta : Outport
  wires:
  abc/1 -> MATLAB Function1/1(u), MATLAB Function/1(u)
  MATLAB Function/1(y) -> Mux/1
  MATLAB Function1/1(y) -> Mux/2
  Mux/1 -> alpha/beta/1

== system dfig(1)/Control1/Angle/abc-->alpha//beta ==
  abc : Inport
  MATLAB Function : MATLAB Function  TreatAsAtomicUnit=on
  MATLAB Function1 : MATLAB Function  TreatAsAtomicUnit=on
  Mux : Mux  Inputs=2
  alpha/beta : Outport
  wires:
  abc/1 -> MATLAB Function1/1(u), MATLAB Function/1(u)
  MATLAB Function/1(y) -> Mux/1
  MATLAB Function1/1(y) -> Mux/2
  Mux/1 -> alpha/beta/1

== matlab function dfig(1)/WT model/MATLAB Function1 ==
  data: u input; y output
function y = fcn(u)
Radio = 42;
y = Radio * (u(2)/u(1))

== matlab function dfig(1)/Control1/Angle/abc-->alpha//beta/MATLAB Function ==
  data: u input; y output
function y = fcn(u)
y=(2/3) * (u(1) - u(2)/2 - u(3)/2);

== matlab function dfig(1)/Control/MPPT/MATLAB Function ==
  data: u input; y output
function y = fcn(u)

y = u(1)*u(1);

== matlab function dfig(1)/Control1/Angle/abc-->alpha//beta/MATLAB Function1 ==
  data: u input; y output
function y = fcn(u)

y=(2/3) * (u(2) * (sqrt(3)/2) - u(3) * (sqrt(3)/2));

== matlab function dfig(1)/Control1/Cancelation of ct/MATLAB Function ==
  data: u input; y output
function y = fcn(u)
Lg = 4.0000e-04;
f = 50;
y = u(1)-u(4)*Lg*(2*pi*f);

== matlab function dfig(1)/Control/DQ-->abc/MATLAB Function ==
  data: u input; y output
function y = fcn(u)
y=u(1);

== matlab function dfig(1)/Control1/Cancelation of ct/MATLAB Function1 ==
  data: u input; y output
function y = fcn(u)
Lg = 40000e-04;
f = 50;
y = u(2)+u(3)*Lg*(2*pi*f);

== matlab function dfig(1)/Control1/alpha//beta->abc/MATLAB Function ==
  data: u input; y output
function y = fcn(u)
y=u(1);

== matlab function dfig(1)/Control1/alpha//beta->abc/MATLAB Function1 ==
  data: u input; y output
function y = fcn(u)
y=-(u(1)/2)+u(2)*(sqrt(3)/2);

== matlab function dfig(1)/Control1/alpha//beta->abc/MATLAB Function2 ==
  data: u input; y output
function y = fcn(u)
y=-(u(1)/2)-u(2)*(sqrt(3)/2);

== matlab function dfig(1)/Control1/abc-->alpha//beta/MATLAB Function ==
  data: u input; y output
function y = fcn(u)

y = (2/3) * (u(1)-u(2)/2-u(3)/2);

== matlab function dfig(1)/Control1/abc-->alpha//beta/MATLAB Function1 ==
  data: u input; y output
function y = fcn(u)

y = (2/3) * (u(2)*(sqrt(3)/2)-u(3)*(sqrt(3)/2));

== matlab function dfig(1)/Control1/d//q-->alpha//beta/MATLAB Function ==
  data: u input; y output
function y = fcn(u)
y=u(1)*cos(u(3))-u(2)*sin(u(3));

== matlab function dfig(1)/Control1/d//q-->alpha//beta/MATLAB Function1 ==
  data: u input; y output
function y = fcn(u)
y=u(1)*sin(u(3))+u(2)*cos(u(3));

== matlab function dfig(1)/Control1/alpha//beta-->d//q/MATLAB Function ==
  data: u input; y output
function y = fcn(u)

y = u(1)*cos(u(3))+u(2)*sin(u(3));

== matlab function dfig(1)/Control1/alpha//beta-->d//q/MATLAB Function1 ==
  data: u input; y output
function y = fcn(u)

y = -u(1)*sin(u(3))+u(2)*cos(u(3));

== matlab function dfig(1)/Control/DQ-->abc/MATLAB Function2 ==
  data: u input; y output
function y = fcn(u)
y=-(u(1)/2)-u(2)*(sqrt(3)/2);

== matlab function dfig(1)/Control/d//q-->D//Q/MATLAB Function ==
  data: u input; y output
function y = fcn(u)
y=u(1)*cos(u(3))-u(2)*sin(u(3));

== matlab function dfig(1)/Control/d//q-->D//Q/MATLAB Function1 ==
  data: u input; y output
function y = fcn(u)
y=u(1)*sin(u(3))+u(2)*cos(u(3));

== matlab function dfig(1)/Control/DQ-->d//q/MATLAB Function ==
  data: u input; y output
function y = fcn(u)

y = u(1)*cos(u(3))+u(2)*sin(u(3));

== matlab function dfig(1)/Control/DQ-->d//q/MATLAB Function1 ==
  data: u input; y output
function y = fcn(u)

y = -u(1)*sin(u(3))+u(2)*cos(u(3));

== matlab function dfig(1)/Control/abc-->DQ/MATLAB Function ==
  data: u input; y output
function y = fcn(u)

y = (2/3) * (u(1)-u(2)/2-u(3)/2);

== matlab function dfig(1)/Control/abc-->DQ/MATLAB Function1 ==
  data: u input; y output
function y = fcn(u)

y = (2/3) * (u(2)*(sqrt(3)/2)-u(3)*(sqrt(3)/2));

== matlab function dfig(1)/Control/DQ-->abc/MATLAB Function1 ==
  data: u input; y output
function y = fcn(u)
y=-(u(1)/2)+u(2)*(sqrt(3)/2);

== matlab function dfig(1)/Control/Angle/abc-->DQ/MATLAB Function ==
  data: u input; y output
function y = fcn(u)
y=(2/3) * (u(1) - u(2)/2 - u(3)/2);

== matlab function dfig(1)/Control/Angle/abc-->DQ/MATLAB Function1 ==
  data: u input; y output
function y = fcn(u)

y=(2/3) * (u(2) * (sqrt(3)/2) - u(3) * (sqrt(3)/2));

== matlab function dfig(1)/Control/Cancelation of cc/MATLAB Function ==
  data: u input; y output
function y = fcn(u)
Lsi = 0.087e-3;
Lm = 2.5e-3;
Ls = Lm + Lsi;
Lr = Lm + Lsi;
sigma = 1 - Lm^2/(Ls*Lr);
y = u(1)-u(5)*sigma*Lr*u(4);

== matlab function dfig(1)/Control/Cancelation of cc/MATLAB Function1 ==
  data: u input; y output
function y = fcn(u)
Lsi = 0.087e-3;
Lm = 2.5e-3;
Ls = Lm + Lsi;
Lr = Lm + Lsi;
sigma = 1 - Lm^2/(Ls*Lr);
y = u(2)+u(5)*sigma*Lr*u(3)*u(5)*(Lm/Ls)*u(6);

== matlab function dfig(1)/WT model/MATLAB Function2 ==
  data: u input; y output
function y = fcn(u)
Radio = 42;
ro = 1.225;
y = (1/2) * ro * pi * (Radio)^3 * (u(2)^2*u(1));
